simulink model "PLL_Sim_Rev5_with_Self_Made_PhaseDetector"  (R2019b)
settings: Solver=VariableStepAuto  StartTime=0.0  StopTime=0.018  MaxStep=100  MinStep=1e-10  RelTol=1e-2  AbsTol=1e-2
libraries: fl_lib x18, ee_lib x13, nesl_utility x7, dspswit3 x2, impairlib x2
settings Model: Creator=connerhannon  LastModifiedBy=connerhannon
settings SolverCC: MaxConsecutiveZCs=100000  MaxConsecutiveMinStep=100000
settings DataIOCC: LimitDataPoints=on  MaxDataPoints=1500

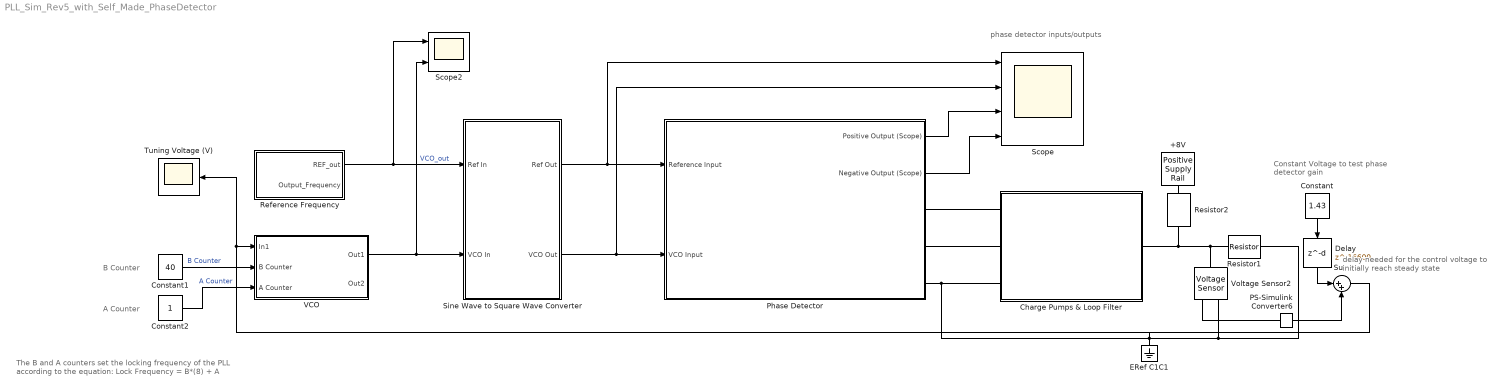
== system PLL_Sim_Rev5_with_Self_Made_PhaseDetector ==
  note: phase detector inputs/outputs
  note: delay needed for the control voltage
      | to initially reach steady state
  note: Constant Voltage to test
      | phase detector gain
  note: A Counter
  note: The B and A counters set the locking frequency of the PLL
      | according to the equation:
      |
      | Lock Frequency = B*(8) + A
  note: B Counter
  "+8V " : ee_lib/Sources/Positive Supply Rail  v0=8 V
      settings: SourceProductName=Simscape Electrical  SourceProductBaseCode=PS  InternalSimscapePortConfiguration="{\"Bottom\":[],\"Left\":[],\"Right\":[{\"id\":\"p\",\"label\":\"\",\"type\":\"foundation.electrical.electrical\"}],\"Top\":[]}"
  Charge Pumps & Loop Filter : Subsystem
  Constant : Constant  Value=1.43
  Constant1 : Constant  Value=40
  Constant2 : Constant
  Delay : Delay  DelayLength=16600  InitialCondition=0
  ERef C1C1 : fl_lib/Electrical/Electrical Elements/Electrical Reference
  PS-Simulink Converter6 : nesl_utility/PS-Simulink Converter  PhysicalDomain=network_engine_domain  SubClassName=ps_output  LeftPortType=input  RightPortType=output  PseudoPeriodic=off  Frequencies=[]  Unit=inherit  AffineConversion=off
  Phase Detector : Subsystem
  Reference Frequency : Subsystem
  Resistor1 : fl_lib/Electrical/Electrical Elements/Resistor  R=10 kOhm  i_specify=off  i_priority=None  i=0 A  i_nominal_specify=off  i_nominal_unit=A  i_nominal_value=1  v_specify=off  v_priority=None  v=0 V  v_nominal_specify=off  v_nominal_unit=V  v_nominal_value=1
  Resistor2 : fl_lib/Electrical/Electrical Elements/Resistor  R=100000 MOhm  i_specify=off  i_priority=None  i=0 A  i_nominal_specify=off  i_nominal_unit=A  i_nominal_value=1  v_specify=off  v_priority=None  v=0 V  v_nominal_specify=off  v_nominal_unit=V  v_nominal_value=1
  Scope : Scope  NumInputPorts=4
  Scope2 : Scope  NumInputPorts=2
  Sine Wave to Square Wave Converter : Subsystem
  Sum : Sum  Inputs=|++
  Tuning Voltage (V) : Scope
  VCO : Subsystem
  Voltage Sensor2 : fl_lib/Electrical/Electrical Sensors/Voltage Sensor
  wires:
  Reference Frequency/1(REF_out) -> Scope2/1, Sine Wave to Square Wave Converter/1(Ref In)
  Constant2/1 -> VCO/3(A Counter)  "A Counter"
  VCO/1(Out1) -> Scope2/2, Sine Wave to Square Wave Converter/2(VCO In)  "VCO_out"
  Constant1/1 -> VCO/2(B Counter)  "B Counter"
  Sine Wave to Square Wave Converter/1(Ref Out) -> Scope/1, Phase Detector/1(Reference Input)
  Sine Wave to Square Wave Converter/2(VCO Out) -> Scope/2, Phase Detector/2(VCO Input)
  Phase Detector/1(Positive Output (Scope)) -> Scope/3
  Phase Detector/2(Negative Output (Scope)) -> Scope/4
  Constant/1 -> Delay/1
  Sum/1 -> Tuning Voltage (V)/1, VCO/1(In1)
  Delay/1 -> Sum/1
  PS-Simulink Converter6/1 -> Sum/2
  connections:
  Voltage Sensor2/RConn1 -- PS-Simulink Converter6/LConn1
  Phase Detector/RConn1 -- Charge Pumps & Loop Filter/LConn1
  Charge Pumps & Loop Filter/LConn2 -- Phase Detector/RConn2
  "+8V "/RConn1 -- Resistor2/LConn1
  ERef C1C1/LConn1 -- Voltage Sensor2/RConn2 -- Resistor1/RConn1 -- Charge Pumps & Loop Filter/LConn3 -- Phase Detector/RConn3
  Resistor2/RConn1 -- Resistor1/LConn1 -- Voltage Sensor2/LConn1 -- Charge Pumps & Loop Filter/RConn1

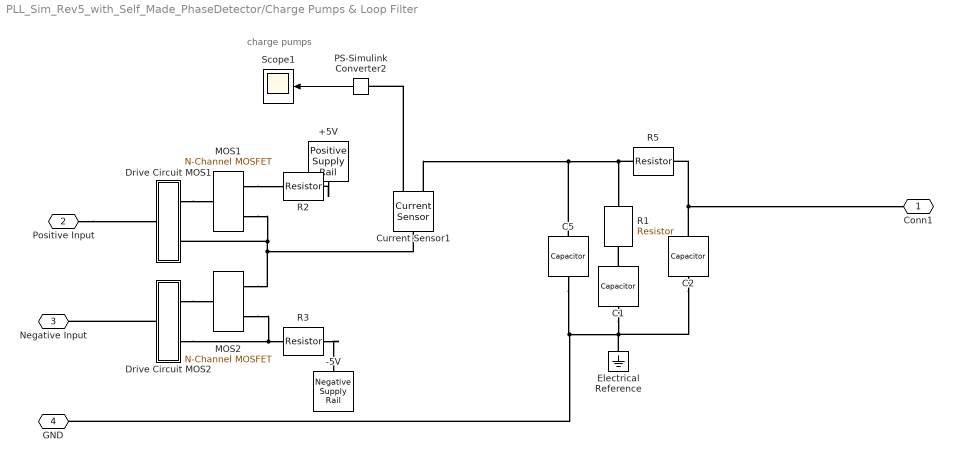
== system PLL_Sim_Rev5_with_Self_Made_PhaseDetector/Charge Pumps & Loop Filter ==
  note: charge pumps
  "+5V " : ee_lib/Sources/Positive Supply Rail  v0=5 V
      settings: SourceProductName=Simscape Electrical  SourceProductBaseCode=PS  InternalSimscapePortConfiguration="{\"Bottom\":[],\"Left\":[],\"Right\":[{\"id\":\"p\",\"label\":\"\",\"type\":\"foundation.electrical.electrical\"}],\"Top\":[]}"
  -5V : ee_lib/Sources/Negative Supply Rail  v0=-5 V
      settings: SourceProductName=Simscape Electrical  SourceProductBaseCode=PS  InternalSimscapePortConfiguration="{\"Bottom\":[],\"Left\":[{\"id\":\"n\",\"label\":\"\",\"type\":\"foundation.electrical.electrical\"}],\"Right\":[],\"Top\":[]}"
  C1 : fl_lib/Electrical/Electrical Elements/Capacitor  c=80 nF  r=1e-6 Ohm  g=0 1/Ohm  i_specify=off  i_priority=High  i=0 A  i_nominal_specify=off  i_nominal_unit=A  i_nominal_value=1  v_specify=off  v_priority=High  v=0 V  v_nominal_specify=off  v_nominal_unit=V  v_nominal_value=1  vc_specify=on  vc_priority=None  vc=0 V  vc_nominal_specify=off  vc_nominal_unit=V  vc_nominal_value=1
  C2 : fl_lib/Electrical/Electrical Elements/Capacitor  c=220 nF  r=1e-6 Ohm  g=0 1/Ohm  i_specify=off  i_priority=High  i=0 A  i_nominal_specify=off  i_nominal_unit=A  i_nominal_value=1  v_specify=off  v_priority=High  v=0 V  v_nominal_specify=off  v_nominal_unit=V  v_nominal_value=1  vc_specify=on  vc_priority=None  vc=0 V  vc_nominal_specify=off  vc_nominal_unit=V  vc_nominal_value=1
  C5 : fl_lib/Electrical/Electrical Elements/Capacitor  c=12 nF  r=1e-6 Ohm  g=0 1/Ohm  i_specify=off  i_priority=High  i=0 A  i_nominal_specify=off  i_nominal_unit=A  i_nominal_value=1  v_specify=off  v_priority=High  v=0 V  v_nominal_specify=off  v_nominal_unit=V  v_nominal_value=1  vc_specify=on  vc_priority=None  vc=0 V  vc_nominal_specify=off  vc_nominal_unit=V  vc_nominal_value=1
  Current Sensor1 : fl_lib/Electrical/Electrical Sensors/Current Sensor
  Drive Circuit MOS1 : Subsystem
  Drive Circuit MOS2 : Subsystem
  Electrical Reference : fl_lib/Electrical/Electrical Elements/Electrical Reference
  MOS1 : ee_lib/Semiconductors & Converters/N-Channel MOSFET  parameterization=1  prmDatasheet=1  prmEquCoeff=1  Beta=5 A/V^2  Rds=1000 Ohm  Id=1e-3 A  Vgs=5 V  Vth=1 V  lam=0 1/V  Tmeas=25 degC  RS=1 Ohm  RD=1 Ohm  C_param=1  C_GS=270 pF  C_GD=80 pF  C_DS=0 pF  C_iss=0.35 pF  C_rss=0.1 pF  C_oss=0 pF  C_GS_vec=[ 270 300 290 280 295 255 ] pF  C_GD_vec=[ 450 400 300 190 95 55 ] pF  C_DS_vec=[ 450 410 390 230 175 115 ] pF  C_iss_vec=[ 720 700 590 470 390 310 ] pF  C_rss_vec=[ 450 400 300 190 95 55 ] pF  C_oss_vec=[ 900 810 690 420 270 170 ] pF  C_Vds_vec=[ 0.1 0.3 1 3 10 30 ] V  V_GS_for_cap_data=NaN V  charge_linearity_param=1  C_OX=200 pF  V_C_OX=-0.5 V  IsDiode=0 A  Vbi=0.6 V  n=1  Cj0Diode=0 pF  TT=50e-9 s  dVth_dT=-6 mV/K  Rds_T2=0.037 Ohm  Tmeas2=125 degC  BEXDatasheet=-1.5  BEXEquCoeff=-1.5  etaisDatasheet=3  etaisEquCoeff=3  TdeviceDatasheet=25 degC  TdeviceEquCoeff=25 degC  thermal_network_parameterization=ee.enum.thermalNetworkTopology.cauer  Rth=[0, 10] K/W  Rth_Foster=[4, 6] K/W  thermal_mass_parameterization=ee.enum.thermalNetwork.timeconstant  thermal_mass=[0, 1] J/K  thermal_mass_Foster=[1.5, 3] J/K  thermal_time_constant=[0, 10] s  thermal_time_constant_Foster=[6, 18] s  thermal_mass_initial_temperatures=[25, 25] degC  betaref=18 A/V^2  Vfbref=-1.1 V  gamma=3.5 V^0.50000  phib2ref=1 V  thesatref=0.4 1/V  alpha=0  Vp=5e-2 V  thesrref=0 1/V  m=8  Tref=25 degC  Cox=1500 pF  Cgso=100 pF  Cgdo=14 pF  Rsref=2e-3 Ohm  Rdref=0.17 Ohm  Rgref=8.4 Ohm  Isref=5.2e-13 A  Cj0=480 pF  Tprm=1  etabet=1.3  Stvfb=5e-4 V/K  Stphib=-8.5e-4 V/K  etasat=1.04  etasr=0.65  etar=0.95  etais=3  Tsim=25 degC  T0=[25, 25] degC
      settings: SourceProductName=Simscape Electrical
  MOS2 : ee_lib/Semiconductors & Converters/N-Channel MOSFET  parameterization=1  prmDatasheet=1  prmEquCoeff=1  Beta=5 A/V^2  Rds=1000 Ohm  Id=1e-3 A  Vgs=5 V  Vth=1 V  lam=0 1/V  Tmeas=25 degC  RS=1 Ohm  RD=1 Ohm  C_param=1  C_GS=270 pF  C_GD=80 pF  C_DS=0 pF  C_iss=0.35 pF  C_rss=0.1 pF  C_oss=0 pF  C_GS_vec=[ 270 300 290 280 295 255 ] pF  C_GD_vec=[ 450 400 300 190 95 55 ] pF  C_DS_vec=[ 450 410 390 230 175 115 ] pF  C_iss_vec=[ 720 700 590 470 390 310 ] pF  C_rss_vec=[ 450 400 300 190 95 55 ] pF  C_oss_vec=[ 900 810 690 420 270 170 ] pF  C_Vds_vec=[ 0.1 0.3 1 3 10 30 ] V  V_GS_for_cap_data=NaN V  charge_linearity_param=1  C_OX=200 pF  V_C_OX=-0.5 V  IsDiode=0 A  Vbi=0.6 V  n=1  Cj0Diode=0 pF  TT=50e-9 s  dVth_dT=-6 mV/K  Rds_T2=0.037 Ohm  Tmeas2=125 degC  BEXDatasheet=-1.5  BEXEquCoeff=-1.5  etaisDatasheet=3  etaisEquCoeff=3  TdeviceDatasheet=25 degC  TdeviceEquCoeff=25 degC  thermal_network_parameterization=ee.enum.thermalNetworkTopology.cauer  Rth=[0, 10] K/W  Rth_Foster=[4, 6] K/W  thermal_mass_parameterization=ee.enum.thermalNetwork.timeconstant  thermal_mass=[0, 1] J/K  thermal_mass_Foster=[1.5, 3] J/K  thermal_time_constant=[0, 10] s  thermal_time_constant_Foster=[6, 18] s  thermal_mass_initial_temperatures=[25, 25] degC  betaref=18 A/V^2  Vfbref=-1.1 V  gamma=3.5 V^0.50000  phib2ref=1 V  thesatref=0.4 1/V  alpha=0  Vp=5e-2 V  thesrref=0 1/V  m=8  Tref=25 degC  Cox=1500 pF  Cgso=100 pF  Cgdo=14 pF  Rsref=2e-3 Ohm  Rdref=0.17 Ohm  Rgref=8.4 Ohm  Isref=5.2e-13 A  Cj0=480 pF  Tprm=1  etabet=1.3  Stvfb=5e-4 V/K  Stphib=-8.5e-4 V/K  etasat=1.04  etasr=0.65  etar=0.95  etais=3  Tsim=25 degC  T0=[25, 25] degC
      settings: SourceProductName=Simscape Electrical
  PS-Simulink Converter2 : nesl_utility/PS-Simulink Converter  PhysicalDomain=network_engine_domain  SubClassName=ps_output  LeftPortType=input  RightPortType=output  PseudoPeriodic=off  Frequencies=[]  Unit=inherit  AffineConversion=off
  R1 : ee_lib/Passive/Resistor  R=62 kOhm  R_tol=5  enable_R_tol=0  tol_distribution=1  nSigma=4  enable_operating_limits=0  operating_limit_action=2  max_working_voltage=100 V  power_rating=1 W  enable_faults=0  fault_action=1  R_faulted=Inf Ohm  enable_temporal_fault=0  t_fault=1 s  enable_behavioral_fault=0  max_permissible_current=1 A  t_fail_on_current=1 s  noise_mode=0  sample_time=0.001 s  repeatability=1  auto_seed=3824493394  user_seed=0  Tdevice=25 degC  alpha=3.93e-3 1/K  Tmeas=25 degC  thermal_mass=100 J/K  power_derating_T1=70 degC  power_derating_T2=155 degC  operating_temperature_range_vec=[-50, 150] degC  temperature_specify=off  temperature_priority=High  temperature=298.15 K  temperature_nominal_specify=off  temperature_nominal_unit=K  temperature_nominal_value=1
      settings: SourceProductName=Simscape Electrical
  R2 : ee_lib/Passive/Resistor  R=5 kOhm  R_tol=5  enable_R_tol=0  tol_distribution=1  nSigma=4  enable_operating_limits=0  operating_limit_action=2  max_working_voltage=100 V  power_rating=1 W  enable_faults=0  fault_action=1  R_faulted=Inf Ohm  enable_temporal_fault=0  t_fault=1 s  enable_behavioral_fault=0  max_permissible_current=1 A  t_fail_on_current=1 s  noise_mode=0  sample_time=0.001 s  repeatability=1  auto_seed=3333544803  user_seed=0  Tdevice=25 degC  alpha=3.93e-3 1/K  Tmeas=25 degC  thermal_mass=100 J/K  power_derating_T1=70 degC  power_derating_T2=155 degC  operating_temperature_range_vec=[-50, 150] degC  temperature_specify=off  temperature_priority=High  temperature=298.15 K  temperature_nominal_specify=off  temperature_nominal_unit=K  temperature_nominal_value=1
      settings: SourceProductName=Simscape Electrical
  R3 : ee_lib/Passive/Resistor  R=5 kOhm  R_tol=5  enable_R_tol=0  tol_distribution=1  nSigma=4  enable_operating_limits=0  operating_limit_action=2  max_working_voltage=100 V  power_rating=1 W  enable_faults=0  fault_action=1  R_faulted=Inf Ohm  enable_temporal_fault=0  t_fault=1 s  enable_behavioral_fault=0  max_permissible_current=1 A  t_fail_on_current=1 s  noise_mode=0  sample_time=0.001 s  repeatability=1  auto_seed=3777182492  user_seed=0  Tdevice=25 degC  alpha=3.93e-3 1/K  Tmeas=25 degC  thermal_mass=100 J/K  power_derating_T1=70 degC  power_derating_T2=155 degC  operating_temperature_range_vec=[-50, 150] degC  temperature_specify=off  temperature_priority=High  temperature=298.15 K  temperature_nominal_specify=off  temperature_nominal_unit=K  temperature_nominal_value=1
      settings: SourceProductName=Simscape Electrical
  R5 : ee_lib/Passive/Resistor  R=1 kOhm  R_tol=5  enable_R_tol=0  tol_distribution=1  nSigma=4  enable_operating_limits=0  operating_limit_action=2  max_working_voltage=100 V  power_rating=1 W  enable_faults=0  fault_action=1  R_faulted=Inf Ohm  enable_temporal_fault=0  t_fault=1 s  enable_behavioral_fault=0  max_permissible_current=1 A  t_fail_on_current=1 s  noise_mode=0  sample_time=0.001 s  repeatability=1  auto_seed=3438132503  user_seed=0  Tdevice=25 degC  alpha=3.93e-3 1/K  Tmeas=25 degC  thermal_mass=100 J/K  power_derating_T1=70 degC  power_derating_T2=155 degC  operating_temperature_range_vec=[-50, 150] degC  temperature_specify=off  temperature_priority=High  temperature=298.15 K  temperature_nominal_specify=off  temperature_nominal_unit=K  temperature_nominal_value=1
      settings: SourceProductName=Simscape Electrical
  Scope1 : Scope
  Conn1 : PMIOPort  Side=Right
  Positive Input : PMIOPort  Port=2  Side=Left
  Negative Input : PMIOPort  Port=3  Side=Left
  GND : PMIOPort  Port=4  Side=Left
  wires:
  PS-Simulink Converter2/1 -> Scope1/1
  connections:
  "+5V "/RConn1 -- R2/LConn1
  C2/LConn1 -- R5/RConn1 -- Conn1/RConn1
  R3/RConn1 -- -5V/LConn1
  MOS2/RConn1 -- Drive Circuit MOS1/RConn2 -- MOS1/RConn2 -- Current Sensor1/LConn1
  Drive Circuit MOS2/RConn1 -- MOS2/LConn1
  Drive Circuit MOS1/RConn1 -- MOS1/LConn1
  Drive Circuit MOS2/LConn1 -- Negative Input/RConn1
  Positive Input/RConn1 -- Drive Circuit MOS1/LConn1
  Drive Circuit MOS2/RConn2 -- R3/LConn1 -- MOS2/RConn2
  C1/LConn1 -- R1/RConn1
  MOS1/RConn1 -- R2/RConn1
  Current Sensor1/RConn1 -- PS-Simulink Converter2/LConn1
  C5/RConn1 -- GND/RConn1 -- Electrical Reference/LConn1 -- C1/RConn1 -- C2/RConn1
  Current Sensor1/RConn2 -- C5/LConn1 -- R5/LConn1 -- R1/LConn1

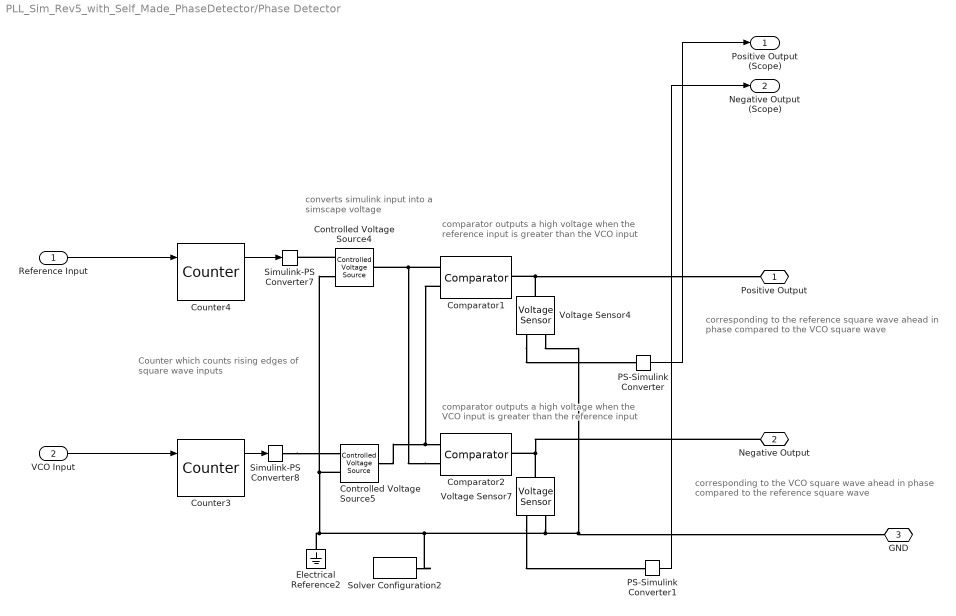
== system PLL_Sim_Rev5_with_Self_Made_PhaseDetector/Phase Detector ==
  note: corresponding to the reference square wave
      | ahead in phase compared to the VCO square wave
  note: comparator outputs a high voltage when the
      | reference input is greater than the VCO input
  note: converts simulink input
      | into a simscape voltage
  note: Counter which counts
      | rising edges of square wave inputs
  note: comparator outputs a high voltage when the
      | VCO input is greater than the reference input
  note: corresponding to the VCO square wave
      | ahead in phase compared to the reference square wave
  Reference Input : Inport
  VCO Input : Inport  Port=2
  Comparator1 : ee_lib/Integrated Circuits/Comparator  V_OS=0 mV  V_OL=0 V  V_OH=5 V  C_IN=0 pF  R_OUT=50 Ohm  Delay=0 s
      settings: SourceProductName=Simscape Electrical  SourceProductBaseCode=PS  InternalSimscapePortConfiguration="{\"Bottom\":[],\"Left\":[{\"id\":\"p\",\"label\":\"+\",\"type\":\"foundation.electrical.electrical\"},{\"id\":\"n\",\"label\":\"-\",\"type\":\"foundation.electrical.electrical\"}],\"Right\":[{\"id\":\"J\",\"label\":\"\",\"type\":\"foundation.electrical.electrical\"}],\"Top\":[]}"
  Comparator2 : ee_lib/Integrated Circuits/Comparator  V_OS=0 mV  V_OL=0 V  V_OH=5 V  C_IN=0 pF  R_OUT=50 Ohm  Delay=0 s
      settings: SourceProductName=Simscape Electrical  SourceProductBaseCode=PS  InternalSimscapePortConfiguration="{\"Bottom\":[],\"Left\":[{\"id\":\"p\",\"label\":\"+\",\"type\":\"foundation.electrical.electrical\"},{\"id\":\"n\",\"label\":\"-\",\"type\":\"foundation.electrical.electrical\"}],\"Right\":[{\"id\":\"J\",\"label\":\"\",\"type\":\"foundation.electrical.electrical\"}],\"Top\":[]}"
  Controlled Voltage Source4 : fl_lib/Electrical/Electrical Sources/Controlled Voltage Source
  Controlled Voltage Source5 : fl_lib/Electrical/Electrical Sources/Controlled Voltage Source
  Counter3 : dspswit3/Counter  Direction=Up  CountEvent=Rising edge  CounterSize=User defined  MaxCount=255  InitialCount=0  Output=Count and Hit  HitValue=32  ResetInput=on  SamplesPerFrame=1  Ts=1  CntDtype=double  HitDtype=Logical
  Counter4 : dspswit3/Counter  Direction=Up  CountEvent=Rising edge  CounterSize=User defined  MaxCount=255  InitialCount=0  Output=Count and Hit  HitValue=32  ResetInput=on  SamplesPerFrame=1  Ts=1  CntDtype=double  HitDtype=Logical
  Electrical Reference2 : fl_lib/Electrical/Electrical Elements/Electrical Reference
  PS-Simulink Converter : nesl_utility/PS-Simulink Converter  PhysicalDomain=network_engine_domain  SubClassName=ps_output  LeftPortType=input  RightPortType=output  PseudoPeriodic=off  Frequencies=[]  Unit=inherit  AffineConversion=off
  PS-Simulink Converter1 : nesl_utility/PS-Simulink Converter  PhysicalDomain=network_engine_domain  SubClassName=ps_output  LeftPortType=input  RightPortType=output  PseudoPeriodic=off  Frequencies=[]  Unit=inherit  AffineConversion=off
  Simulink-PS Converter7 : nesl_utility/Simulink-PS Converter  PhysicalDomain=network_engine_domain  SubClassName=ps_input  LeftPortType=input  RightPortType=output  PseudoPeriodic=off  Frequencies=[]  NoiseDistribution=none  NoiseParameters=[]  Unit=1  AffineConversion=off  FilteringAndDerivatives=provide  SimscapeFilterOrder=1  InputFilterTimeConstant=0.001  UdotUserProvided=0
  Simulink-PS Converter8 : nesl_utility/Simulink-PS Converter  PhysicalDomain=network_engine_domain  SubClassName=ps_input  LeftPortType=input  RightPortType=output  PseudoPeriodic=off  Frequencies=[]  NoiseDistribution=none  NoiseParameters=[]  Unit=1  AffineConversion=off  FilteringAndDerivatives=provide  SimscapeFilterOrder=1  InputFilterTimeConstant=0.001  UdotUserProvided=0
  Solver Configuration2 : nesl_utility/Solver Configuration  PhysicalDomain=network_engine_domain  SubClassName=solver  LeftPortType=input  RightPortType=generic  Tones=[]  Harmonics=[]  SimulateNoise=off  Profile=off  UseLocalSampling=off  EnableSwitchedLinearOptims=on  FrequencyDomain=off  UseCCode=off  RelTol=0.001  AbsTol=1e-06  MinStep=1e-09  ToWorkspace=off  RevertToSquareIcSolve=off  NumHomotopyIterations=100  PhasorMode=off  PhasorModeNumHarmonics=1  DoDC=off  ResidualTolerance=1e-6  UseLocalSolver=off  LocalSolverChoice=NE_TRAPEZOIDAL_ADVANCER  LocalSolverSampleTime=1e-9  DoFixedCost=off  MaxNonlinIter=3  MaxModeIter=2  LinearAlgebra=auto  EquationFormulation=NE_TIME_EF  DelaysMemoryBudget=1024  AutomaticFiltering=on  FilteringTimeConstant=0.0001  PartitionStorageMethod=AS_NEEDED  PartitionMemoryBudget=1024  PartitionMethod=FAST
  Voltage Sensor4 : fl_lib/Electrical/Electrical Sensors/Voltage Sensor
  Voltage Sensor7 : fl_lib/Electrical/Electrical Sensors/Voltage Sensor
  Positive Output : PMIOPort  Side=Right
  Negative Output : PMIOPort  Port=2  Side=Right
  GND : PMIOPort  Port=3  Side=Right
  Positive Output (Scope) : Outport
  Negative Output (Scope) : Outport  Port=2
  wires:
  PS-Simulink Converter/1 -> Positive Output (Scope)/1
  VCO Input/1 -> Counter3/1
  PS-Simulink Converter1/1 -> Negative Output (Scope)/1
  Counter3/1 -> Simulink-PS Converter8/1
  Counter4/1 -> Simulink-PS Converter7/1
  Reference Input/1 -> Counter4/1
  connections:
  Simulink-PS Converter8/RConn1 -- Controlled Voltage Source5/RConn1
  Controlled Voltage Source4/RConn1 -- Simulink-PS Converter7/RConn1
  Voltage Sensor4/LConn1 -- Comparator1/RConn1 -- Positive Output/RConn1
  Comparator2/LConn1 -- Controlled Voltage Source5/LConn1 -- Comparator1/LConn2
  Voltage Sensor4/RConn1 -- PS-Simulink Converter/LConn1
  Voltage Sensor7/LConn1 -- Negative Output/RConn1 -- Comparator2/RConn1
  Voltage Sensor4/RConn2 -- Solver Configuration2/RConn1 -- Controlled Voltage Source4/RConn2 -- Controlled Voltage Source5/RConn2 -- Electrical Reference2/LConn1 -- Voltage Sensor7/RConn2 -- GND/RConn1
  Voltage Sensor7/RConn1 -- PS-Simulink Converter1/LConn1
  Comparator2/LConn2 -- Controlled Voltage Source4/LConn1 -- Comparator1/LConn1

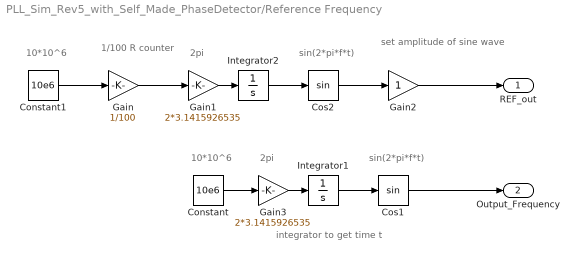
== system PLL_Sim_Rev5_with_Self_Made_PhaseDetector/Reference Frequency ==
  note: 10*10^6
  note: set amplitude of sine wave
  note: 1/100
      | R counter
  note: integrator to get time t
  note: sin(2*pi*f*t)
  note: 2pi
  note: sin(2*pi*f*t)
  note: 2pi
  note: 10*10^6
  Constant : Constant  Value=10e6
  Constant1 : Constant  Value=10e6
  Cos1 : Trigonometry  OutputSignalType=real
  Cos2 : Trigonometry  OutputSignalType=real
  Gain : Gain  Gain=1/100
  Gain1 : Gain  Gain=2*3.1415926535
  Gain2 : Gain
  Gain3 : Gain  Gain=2*3.1415926535
  Integrator1 : Integrator
  Integrator2 : Integrator
  REF_out : Outport
  "Output_Frequency " : Outport  Port=2
  wires:
  Cos1/1 -> "Output_Frequency "/1
  Gain3/1 -> Integrator1/1
  Integrator1/1 -> Cos1/1
  Constant/1 -> Gain3/1
  Constant1/1 -> Gain/1
  Gain1/1 -> Integrator2/1
  Integrator2/1 -> Cos2/1
  Gain/1 -> Gain1/1
  Cos2/1 -> Gain2/1
  Gain2/1 -> REF_out/1

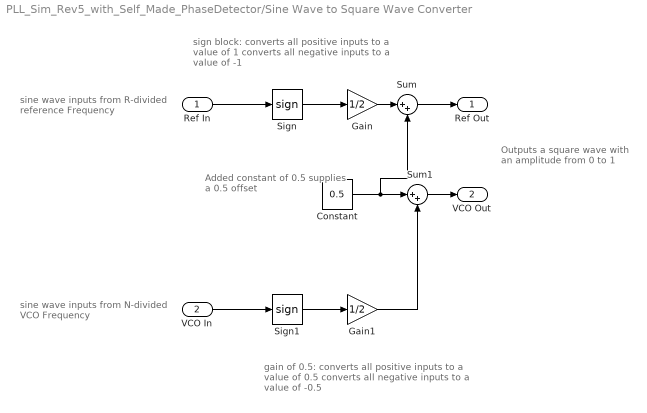
== system PLL_Sim_Rev5_with_Self_Made_PhaseDetector/Sine Wave to Square Wave Converter ==
  note: Outputs a square wave with
      | an amplitude from 0 to 1
  note: Added constant of 0.5
      | supplies a 0.5 offset
  note: gain of 0.5:
      | converts all positive inputs to a value of 0.5
      | converts all negative inputs to a value of -0.5
  note: sign block:
      | converts all positive inputs to a value of 1
      | converts all negative inputs to a value of -1
  note: sine wave inputs from R-divided
      | reference Frequency
  note: sine wave inputs from N-divided
      | VCO Frequency
  Ref In : Inport
  VCO In : Inport  Port=2
  Constant : Constant  Value=0.5
  Gain : Gain  Gain=1/2
  Gain1 : Gain  Gain=1/2
  Sign : Signum
  Sign1 : Signum
  Sum : Sum  Inputs=|++
  Sum1 : Sum  Inputs=|++
  Ref Out : Outport
  VCO Out : Outport  Port=2
  wires:
  Sum/1 -> Ref Out/1
  Sum1/1 -> VCO Out/1
  Gain/1 -> Sum/1
  VCO In/1 -> Sign1/1
  Constant/1 -> Sum1/1, Sum/2
  Sign/1 -> Gain/1
  Sign1/1 -> Gain1/1
  Ref In/1 -> Sign/1
  Gain1/1 -> Sum1/2

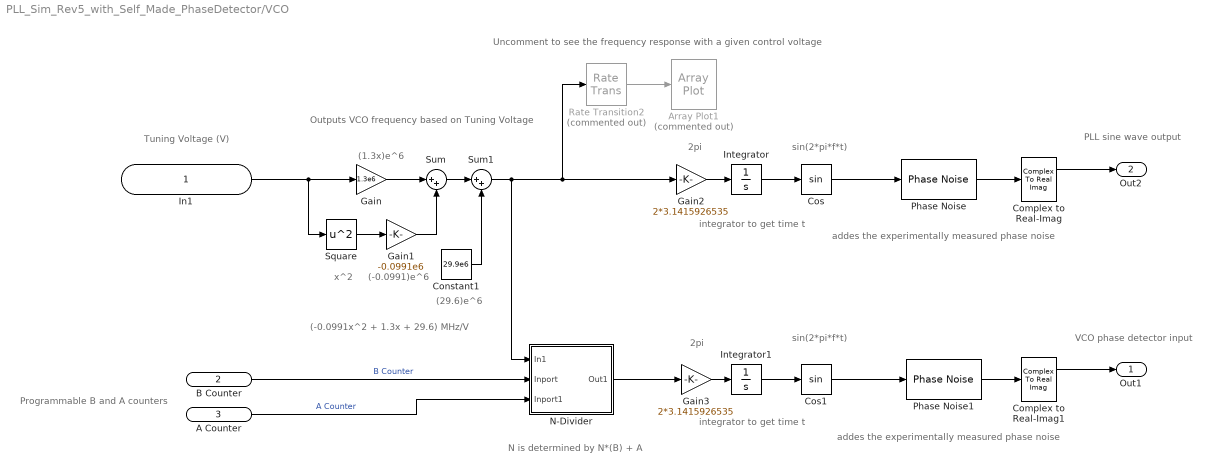
== system PLL_Sim_Rev5_with_Self_Made_PhaseDetector/VCO ==
  note: (29.6)e^6
  note: x^2
  note: (1.3x)e^6
  note: VCO phase detector input
  note: PLL sine wave output
  note: N is determined by N*(B) + A
  note: Programmable B and A counters
  note: Uncomment to see the frequency response with a given control voltage
  note: Tuning Voltage
      | (V)
  note: 2pi
  note: sin(2*pi*f*t)
  note: integrator to get time t
  note: (-0.0991x^2 + 1.3x + 29.6) MHz/V
  note: addes the experimentally measured phase noise
  note: Outputs VCO frequency based on Tuning Voltage
  note: 2pi
  note: integrator to get time t
  note: sin(2*pi*f*t)
  note: addes the experimentally measured phase noise
  note: (-0.0991)e^6
  In1 : Inport
  B Counter : Inport  Port=2
  A Counter : Inport  Port=3
  Array Plot1 : ArrayPlot  Commented=on
  Complex to Real-Imag : ComplexToRealImag
  Complex to Real-Imag1 : ComplexToRealImag
  Constant1 : Constant  Value=29.9e6
  Cos : Trigonometry  OutputSignalType=complex
  Cos1 : Trigonometry  OutputSignalType=complex
  Gain : Gain  Gain=1.3e6
  Gain1 : Gain  Gain=-0.0991e6
  Gain2 : Gain  Gain=2*3.1415926535
  Gain3 : Gain  Gain=2*3.1415926535
  Integrator : Integrator
  Integrator1 : Integrator
  N-Divider : Subsystem
  Phase Noise : impairlib/Phase Noise  Level=[ -36, -73, -83, -90, -112 ]  FrequencyOffset=[ 100, 400, 1000, 5000, 250000]  SampleRate=550000  RandomStream=mt19937ar with seed  Seed=1e6  SimulateUsing=Interpreted execution
      settings: SourceProductName=SerDes Toolbox  SourceProductBaseCode=SX
  Phase Noise1 : impairlib/Phase Noise  Level=[ -36, -73, -83, -90, -112 ]  FrequencyOffset=[ 100, 400, 1000, 5000, 250000]  SampleRate=550000  RandomStream=mt19937ar with seed  Seed=1e6  SimulateUsing=Interpreted execution
      settings: SourceProductName=SerDes Toolbox  SourceProductBaseCode=SX
  Rate Transition2 : RateTransition  Commented=on  OutPortSampleTime=1/1000000000
  Square : Math  Operator=square  SignedPower=off  SaturateOnIntegerOverflow=on
  Sum : Sum  Inputs=|++
  Sum1 : Sum  Inputs=|++
  Out1 : Outport
  Out2 : Outport  Port=2
  wires:
  Gain1/1 -> Sum/2
  Gain/1 -> Sum/1
  Square/1 -> Gain1/1
  Integrator/1 -> Cos/1
  Constant1/1 -> Sum1/2
  Phase Noise/1 -> Complex to Real-Imag/1
  Sum/1 -> Sum1/1
  Cos/1 -> Phase Noise/1
  In1/1 -> Square/1, Gain/1
  Gain2/1 -> Integrator/1
  Gain3/1 -> Integrator1/1
  Phase Noise1/1 -> Complex to Real-Imag1/1
  Integrator1/1 -> Cos1/1
  Complex to Real-Imag1/1 -> Out1/1
  Complex to Real-Imag/1 -> Out2/1
  Cos1/1 -> Phase Noise1/1
  Sum1/1 -> N-Divider/1(In1), Rate Transition2/1, Gain2/1
  B Counter/1 -> N-Divider/2(Inport)  "B Counter"
  A Counter/1 -> N-Divider/3(Inport1)  "A Counter"
  N-Divider/1(Out1) -> Gain3/1
  Rate Transition2/1 -> Array Plot1/1

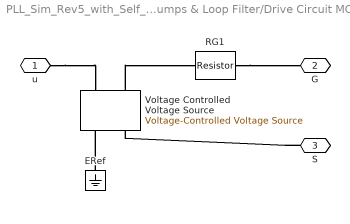
== system PLL_Sim_Rev5_with_Self_Made_PhaseDetector/Charge Pumps & Loop Filter/Drive Circuit MOS1 ==
  ERef : fl_lib/Electrical/Electrical Elements/Electrical Reference
  RG1 : ee_lib/Passive/Resistor  R=40 kOhm  R_tol=5  enable_R_tol=0  tol_distribution=1  nSigma=4  enable_operating_limits=0  operating_limit_action=2  max_working_voltage=100 V  power_rating=1 W  enable_faults=0  fault_action=1  R_faulted=Inf Ohm  enable_temporal_fault=0  t_fault=1 s  enable_behavioral_fault=0  max_permissible_current=1 A  t_fail_on_current=1 s  noise_mode=0  sample_time=0.001 s  repeatability=1  auto_seed=960529170  user_seed=0  Tdevice=25 degC  alpha=3.93e-3 1/K  Tmeas=25 degC  thermal_mass=100 J/K  power_derating_T1=70 degC  power_derating_T2=155 degC  operating_temperature_range_vec=[-50, 150] degC  temperature_specify=off  temperature_priority=High  temperature=298.15 K  temperature_nominal_specify=off  temperature_nominal_unit=K  temperature_nominal_value=1
      settings: SourceProductName=Simscape Electrical
  Voltage Controlled Voltage Source : fl_lib/Electrical/Electrical Sources/Voltage-Controlled Voltage Source  K=1  v1_specify=off  v1_priority=High  v1=0 V  v1_nominal_specify=off  v1_nominal_unit=V  v1_nominal_value=1  v2_specify=off  v2_priority=High  v2=0 V  v2_nominal_specify=off  v2_nominal_unit=V  v2_nominal_value=1
      settings: SourceProductName=Simscape  SourceProductBaseCode=SS  InternalSimscapePortConfiguration="{\"Bottom\":[],\"Left\":[{\"id\":\"p1\",\"label\":\"+\",\"type\":\"foundation.electrical.electrical\"},{\"id\":\"p2\",\"label\":\"+\",\"type\":\"foundation.electrical.electrical\"}],\"Right\":[{\"id\":\"n1\",\"label\":\"-\",\"type\":\"foundation.electrical.electrical\"},{\"id\":\"n2\",\"label\":\"-\",\"type\":\"foundation.electrical.electrical\"}],\"Top\":[]}"
  u : PMIOPort  Side=Left
  G : PMIOPort  Port=2  Side=Right
  S : PMIOPort  Port=3  Side=Right
  connections:
  u/RConn1 -- Voltage Controlled Voltage Source/LConn1
  S/RConn1 -- Voltage Controlled Voltage Source/RConn2
  RG1/RConn1 -- G/RConn1
  Voltage Controlled Voltage Source/LConn2 -- RG1/LConn1
  ERef/LConn1 -- Voltage Controlled Voltage Source/RConn1

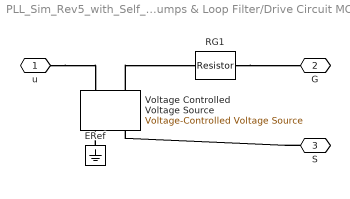
== system PLL_Sim_Rev5_with_Self_Made_PhaseDetector/Charge Pumps & Loop Filter/Drive Circuit MOS2 ==
  ERef : fl_lib/Electrical/Electrical Elements/Electrical Reference
  RG1 : ee_lib/Passive/Resistor  R=40 kOhm  R_tol=5  enable_R_tol=0  tol_distribution=1  nSigma=4  enable_operating_limits=0  operating_limit_action=2  max_working_voltage=100 V  power_rating=1 W  enable_faults=0  fault_action=1  R_faulted=Inf Ohm  enable_temporal_fault=0  t_fault=1 s  enable_behavioral_fault=0  max_permissible_current=1 A  t_fail_on_current=1 s  noise_mode=0  sample_time=0.001 s  repeatability=1  auto_seed=691217465  user_seed=0  Tdevice=25 degC  alpha=3.93e-3 1/K  Tmeas=25 degC  thermal_mass=100 J/K  power_derating_T1=70 degC  power_derating_T2=155 degC  operating_temperature_range_vec=[-50, 150] degC  temperature_specify=off  temperature_priority=High  temperature=298.15 K  temperature_nominal_specify=off  temperature_nominal_unit=K  temperature_nominal_value=1
      settings: SourceProductName=Simscape Electrical
  Voltage Controlled Voltage Source : fl_lib/Electrical/Electrical Sources/Voltage-Controlled Voltage Source  K=1  v1_specify=off  v1_priority=High  v1=0 V  v1_nominal_specify=off  v1_nominal_unit=V  v1_nominal_value=1  v2_specify=off  v2_priority=High  v2=0 V  v2_nominal_specify=off  v2_nominal_unit=V  v2_nominal_value=1
      settings: SourceProductName=Simscape  SourceProductBaseCode=SS  InternalSimscapePortConfiguration="{\"Bottom\":[],\"Left\":[{\"id\":\"p1\",\"label\":\"+\",\"type\":\"foundation.electrical.electrical\"},{\"id\":\"p2\",\"label\":\"+\",\"type\":\"foundation.electrical.electrical\"}],\"Right\":[{\"id\":\"n1\",\"label\":\"-\",\"type\":\"foundation.electrical.electrical\"},{\"id\":\"n2\",\"label\":\"-\",\"type\":\"foundation.electrical.electrical\"}],\"Top\":[]}"
  u : PMIOPort  Side=Left
  G : PMIOPort  Port=2  Side=Right
  S : PMIOPort  Port=3  Side=Right
  connections:
  ERef/LConn1 -- Voltage Controlled Voltage Source/RConn1
  Voltage Controlled Voltage Source/LConn2 -- RG1/LConn1
  RG1/RConn1 -- G/RConn1
  S/RConn1 -- Voltage Controlled Voltage Source/RConn2
  u/RConn1 -- Voltage Controlled Voltage Source/LConn1

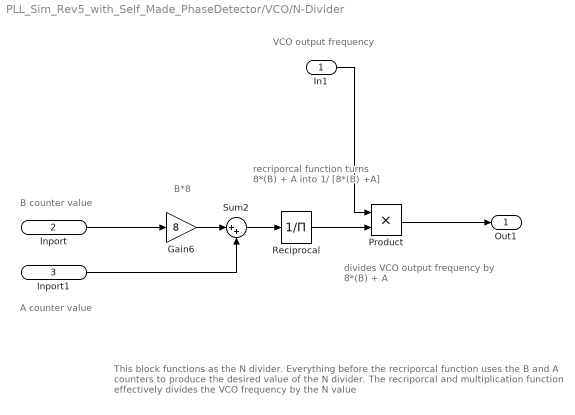
== system PLL_Sim_Rev5_with_Self_Made_PhaseDetector/VCO/N-Divider ==
  note: This block functions as the N divider. Everything before the recriporcal
      | function uses the B and A counters to produce the desired value of the
      | N divider. The recriporcal and multiplication function effectively divides
      | the VCO frequency by the N value
  note: divides VCO output frequency by
      | 8*(B) + A
  note: VCO output frequency
  note: recriporcal function
      | turns 8*(B) + A
      | into  1/ [8*(B) +A]
  note: B*8
  note: A counter value
  note: B counter value
  In1 : Inport
  Inport : Inport  Port=2
  Inport1 : Inport  Port=3
  Gain6 : Gain  Gain=8
  Product : Product
  Reciprocal : Product  Inputs=/
  Sum2 : Sum  Inputs=|++
  Out1 : Outport
  wires:
  Product/1 -> Out1/1
  Inport/1 -> Gain6/1
  Sum2/1 -> Reciprocal/1
  Gain6/1 -> Sum2/1
  Reciprocal/1 -> Product/2
  In1/1 -> Product/1
  Inport1/1 -> Sum2/2
